simulink model "Feeder_1"  (Simulink 8.8)
settings: Solver=ode4  StartTime=0.0  StopTime=inf  FixedStep=Ts  RelTol=1e-3  EnableMultiTasking=on
PreLoadFcn:
  | Ts=125e-6;Core_Num = 0; np=1; nq=1; Vmin=.9;
PostLoadFcn:
  | Ts=125e-6;Core_Num = 0; np=1; nq=1; Vmin=.9;
InitFcn:
  | Ts=125e-6;Core_Num = 0; np=1; nq=1; Vmin=.9;
undefined symbols (not defined in the file or in its folder): another_event_name, DiscIntNeverNeededParam, I, j, Left, my_event_name, Right, type, V, X
libraries: powerlib x316, powerlib_meascontrol x227, simulink_extras x78, simulink x25, rtio_generic_c37_118 x22, ssn_lib x9, rtlab x6, powerlib_extras x3, artemis x1, rtio_opalrt_ml605ex1 x1, rtio_spectracom x1, rtio_generic_ethernet x1
(part 6 of 14)

== system Feeder_1/SM_NG/Single-Phase Dynamic Load43/model ==
  v : Inport
  PQ : Inport  Port=2
  -Q : Gain  SaturateOnIntegerOverflow=on  OutDataTypeStr=Inherit: Same as input  ParamDataTypeStr=Inherit: Same as input
  Break  Alg. Loop1 : Subsystem
  Complex to Magnitude-Angle : ComplexToMagnitudeAngle
  Complex to Real-Imag1 : ComplexToRealImag
  Constant : Constant
  Demux : Demux  Outputs=2
  Divide : Product  Inputs=**
  Gain : Gain  Gain=1.0114
  IC1 : InitialCondition
  IC2 : InitialCondition
  Magnitude-Angle to Complex : MagnitudeAngleToComplex
  PLL : Subsystem  mask{freq=fnom}
      mask prompts: freq "Initial frequency (Hz)"
  Positive Sequence  current : Subsystem
  RMS1 : powerlib_meascontrol/Measurements/RMS  TrueRMS=on  Freq=fnom  RMSInit=1  Ts=0
  Real-Imag to Complex : RealImagToComplex
  Real-Imag to Complex1 : RealImagToComplex
  Sum : Sum
  Transfer Fcn1 : TransferFcn  Numerator=[1 290.1]  Denominator=[1 298.8]
  Trigonometric Function1 : Trigonometry
  V> pu : Gain  Gain=1/Vbase/sqrt(3)  SaturateOnIntegerOverflow=on  OutDataTypeStr=Inherit: Same as input  ParamDataTypeStr=Inherit: Same as input
  V> pu1 : Gain  Gain=sqrt(2)  SaturateOnIntegerOverflow=on  OutDataTypeStr=Inherit: Same as input  ParamDataTypeStr=Inherit: Same as input
  i : Outport
  wires:
  V> pu/1 -> PLL/1(v (pu)), V> pu1/1
  Real-Imag to Complex/1 -> Positive Sequence  current/1(V1(pu))
  PQ/1 -> Demux/1
  Demux/1 -> Real-Imag to Complex1/1
  Demux/2 -> -Q/1
  Real-Imag to Complex1/1 -> Positive Sequence  current/2(S_ext)
  Complex to Real-Imag1/1 -> Real-Imag to Complex/1
  Complex to Real-Imag1/2 -> Real-Imag to Complex/2
  Magnitude-Angle to Complex/1 -> Complex to Real-Imag1/1
  Constant/1 -> PLL/2(freq (pu))
  PLL/1(alpha (rad)) -> Magnitude-Angle to Complex/2
  Complex to Magnitude-Angle/2 -> Sum/2
  PLL/2(wt) -> Sum/1
  Sum/1 -> Trigonometric Function1/1
  Trigonometric Function1/1 -> Divide/2
  Complex to Magnitude-Angle/1 -> Divide/1
  RMS1/1 -> IC1/1
  V> pu1/1 -> RMS1/1
  v/1 -> IC2/1
  Positive Sequence  current/1(I1(A)) -> Break  Alg. Loop1/1(In)
  Break  Alg. Loop1/1(Out) -> Complex to Magnitude-Angle/1
  IC1/1 -> Magnitude-Angle to Complex/1
  IC2/1 -> V> pu/1
  Transfer Fcn1/1 -> Gain/1
  Gain/1 -> i/1
  Divide/1 -> Transfer Fcn1/1
  -Q/1 -> Real-Imag to Complex1/2

== system Feeder_1/SM_NG/Single-Phase Dynamic Load44/model ==
  v : Inport
  PQ : Inport  Port=2
  -Q : Gain  SaturateOnIntegerOverflow=on  OutDataTypeStr=Inherit: Same as input  ParamDataTypeStr=Inherit: Same as input
  Break  Alg. Loop1 : Subsystem
  Complex to Magnitude-Angle : ComplexToMagnitudeAngle
  Complex to Real-Imag1 : ComplexToRealImag
  Constant : Constant
  Demux : Demux  Outputs=2
  Divide : Product  Inputs=**
  Gain : Gain  Gain=1.0114
  IC1 : InitialCondition
  IC2 : InitialCondition
  Magnitude-Angle to Complex : MagnitudeAngleToComplex
  PLL : Subsystem  mask{freq=fnom}
      mask prompts: freq "Initial frequency (Hz)"
  Positive Sequence  current : Subsystem
  RMS1 : powerlib_meascontrol/Measurements/RMS  TrueRMS=on  Freq=fnom  RMSInit=1  Ts=0
  Real-Imag to Complex : RealImagToComplex
  Real-Imag to Complex1 : RealImagToComplex
  Sum : Sum
  Transfer Fcn1 : TransferFcn  Numerator=[1 290.1]  Denominator=[1 298.8]
  Trigonometric Function1 : Trigonometry
  V> pu : Gain  Gain=1/Vbase/sqrt(3)  SaturateOnIntegerOverflow=on  OutDataTypeStr=Inherit: Same as input  ParamDataTypeStr=Inherit: Same as input
  V> pu1 : Gain  Gain=sqrt(2)  SaturateOnIntegerOverflow=on  OutDataTypeStr=Inherit: Same as input  ParamDataTypeStr=Inherit: Same as input
  i : Outport
  wires:
  V> pu/1 -> PLL/1(v (pu)), V> pu1/1
  Real-Imag to Complex/1 -> Positive Sequence  current/1(V1(pu))
  PQ/1 -> Demux/1
  Demux/1 -> Real-Imag to Complex1/1
  Demux/2 -> -Q/1
  Real-Imag to Complex1/1 -> Positive Sequence  current/2(S_ext)
  Complex to Real-Imag1/1 -> Real-Imag to Complex/1
  Complex to Real-Imag1/2 -> Real-Imag to Complex/2
  Magnitude-Angle to Complex/1 -> Complex to Real-Imag1/1
  Constant/1 -> PLL/2(freq (pu))
  PLL/1(alpha (rad)) -> Magnitude-Angle to Complex/2
  Complex to Magnitude-Angle/2 -> Sum/2
  PLL/2(wt) -> Sum/1
  Sum/1 -> Trigonometric Function1/1
  Trigonometric Function1/1 -> Divide/2
  Complex to Magnitude-Angle/1 -> Divide/1
  RMS1/1 -> IC1/1
  V> pu1/1 -> RMS1/1
  v/1 -> IC2/1
  Positive Sequence  current/1(I1(A)) -> Break  Alg. Loop1/1(In)
  Break  Alg. Loop1/1(Out) -> Complex to Magnitude-Angle/1
  IC1/1 -> Magnitude-Angle to Complex/1
  IC2/1 -> V> pu/1
  Transfer Fcn1/1 -> Gain/1
  Gain/1 -> i/1
  Divide/1 -> Transfer Fcn1/1
  -Q/1 -> Real-Imag to Complex1/2

== system Feeder_1/SM_NG/Single-Phase Dynamic Load45/model ==
  v : Inport
  PQ : Inport  Port=2
  -Q : Gain  SaturateOnIntegerOverflow=on  OutDataTypeStr=Inherit: Same as input  ParamDataTypeStr=Inherit: Same as input
  Break  Alg. Loop1 : Subsystem
  Complex to Magnitude-Angle : ComplexToMagnitudeAngle
  Complex to Real-Imag1 : ComplexToRealImag
  Constant : Constant
  Demux : Demux  Outputs=2
  Divide : Product  Inputs=**
  Gain : Gain  Gain=1.0114
  IC1 : InitialCondition
  IC2 : InitialCondition
  Magnitude-Angle to Complex : MagnitudeAngleToComplex
  PLL : Subsystem  mask{freq=fnom}
      mask prompts: freq "Initial frequency (Hz)"
  Positive Sequence  current : Subsystem
  RMS1 : powerlib_meascontrol/Measurements/RMS  TrueRMS=on  Freq=fnom  RMSInit=1  Ts=0
  Real-Imag to Complex : RealImagToComplex
  Real-Imag to Complex1 : RealImagToComplex
  Sum : Sum
  Transfer Fcn1 : TransferFcn  Numerator=[1 290.1]  Denominator=[1 298.8]
  Trigonometric Function1 : Trigonometry
  V> pu : Gain  Gain=1/Vbase/sqrt(3)  SaturateOnIntegerOverflow=on  OutDataTypeStr=Inherit: Same as input  ParamDataTypeStr=Inherit: Same as input
  V> pu1 : Gain  Gain=sqrt(2)  SaturateOnIntegerOverflow=on  OutDataTypeStr=Inherit: Same as input  ParamDataTypeStr=Inherit: Same as input
  i : Outport
  wires:
  V> pu/1 -> PLL/1(v (pu)), V> pu1/1
  Real-Imag to Complex/1 -> Positive Sequence  current/1(V1(pu))
  PQ/1 -> Demux/1
  Demux/1 -> Real-Imag to Complex1/1
  Demux/2 -> -Q/1
  Real-Imag to Complex1/1 -> Positive Sequence  current/2(S_ext)
  Complex to Real-Imag1/1 -> Real-Imag to Complex/1
  Complex to Real-Imag1/2 -> Real-Imag to Complex/2
  Magnitude-Angle to Complex/1 -> Complex to Real-Imag1/1
  Constant/1 -> PLL/2(freq (pu))
  PLL/1(alpha (rad)) -> Magnitude-Angle to Complex/2
  Complex to Magnitude-Angle/2 -> Sum/2
  PLL/2(wt) -> Sum/1
  Sum/1 -> Trigonometric Function1/1
  Trigonometric Function1/1 -> Divide/2
  Complex to Magnitude-Angle/1 -> Divide/1
  RMS1/1 -> IC1/1
  V> pu1/1 -> RMS1/1
  v/1 -> IC2/1
  Positive Sequence  current/1(I1(A)) -> Break  Alg. Loop1/1(In)
  Break  Alg. Loop1/1(Out) -> Complex to Magnitude-Angle/1
  IC1/1 -> Magnitude-Angle to Complex/1
  IC2/1 -> V> pu/1
  Transfer Fcn1/1 -> Gain/1
  Gain/1 -> i/1
  Divide/1 -> Transfer Fcn1/1
  -Q/1 -> Real-Imag to Complex1/2

== system Feeder_1/SM_NG/Single-Phase Dynamic Load46/model ==
  v : Inport
  PQ : Inport  Port=2
  -Q : Gain  SaturateOnIntegerOverflow=on  OutDataTypeStr=Inherit: Same as input  ParamDataTypeStr=Inherit: Same as input
  Break  Alg. Loop1 : Subsystem
  Complex to Magnitude-Angle : ComplexToMagnitudeAngle
  Complex to Real-Imag1 : ComplexToRealImag
  Constant : Constant
  Demux : Demux  Outputs=2
  Divide : Product  Inputs=**
  Gain : Gain  Gain=1.0114
  IC1 : InitialCondition
  IC2 : InitialCondition
  Magnitude-Angle to Complex : MagnitudeAngleToComplex
  PLL : Subsystem  mask{freq=fnom}
      mask prompts: freq "Initial frequency (Hz)"
  Positive Sequence  current : Subsystem
  RMS1 : powerlib_meascontrol/Measurements/RMS  TrueRMS=on  Freq=fnom  RMSInit=1  Ts=0
  Real-Imag to Complex : RealImagToComplex
  Real-Imag to Complex1 : RealImagToComplex
  Sum : Sum
  Transfer Fcn1 : TransferFcn  Numerator=[1 290.1]  Denominator=[1 298.8]
  Trigonometric Function1 : Trigonometry
  V> pu : Gain  Gain=1/Vbase/sqrt(3)  SaturateOnIntegerOverflow=on  OutDataTypeStr=Inherit: Same as input  ParamDataTypeStr=Inherit: Same as input
  V> pu1 : Gain  Gain=sqrt(2)  SaturateOnIntegerOverflow=on  OutDataTypeStr=Inherit: Same as input  ParamDataTypeStr=Inherit: Same as input
  i : Outport
  wires:
  V> pu/1 -> PLL/1(v (pu)), V> pu1/1
  Real-Imag to Complex/1 -> Positive Sequence  current/1(V1(pu))
  PQ/1 -> Demux/1
  Demux/1 -> Real-Imag to Complex1/1
  Demux/2 -> -Q/1
  Real-Imag to Complex1/1 -> Positive Sequence  current/2(S_ext)
  Complex to Real-Imag1/1 -> Real-Imag to Complex/1
  Complex to Real-Imag1/2 -> Real-Imag to Complex/2
  Magnitude-Angle to Complex/1 -> Complex to Real-Imag1/1
  Constant/1 -> PLL/2(freq (pu))
  PLL/1(alpha (rad)) -> Magnitude-Angle to Complex/2
  Complex to Magnitude-Angle/2 -> Sum/2
  PLL/2(wt) -> Sum/1
  Sum/1 -> Trigonometric Function1/1
  Trigonometric Function1/1 -> Divide/2
  Complex to Magnitude-Angle/1 -> Divide/1
  RMS1/1 -> IC1/1
  V> pu1/1 -> RMS1/1
  v/1 -> IC2/1
  Positive Sequence  current/1(I1(A)) -> Break  Alg. Loop1/1(In)
  Break  Alg. Loop1/1(Out) -> Complex to Magnitude-Angle/1
  IC1/1 -> Magnitude-Angle to Complex/1
  IC2/1 -> V> pu/1
  Transfer Fcn1/1 -> Gain/1
  Gain/1 -> i/1
  Divide/1 -> Transfer Fcn1/1
  -Q/1 -> Real-Imag to Complex1/2

== system Feeder_1/SM_NG/Single-Phase Dynamic Load47/model ==
  v : Inport
  PQ : Inport  Port=2
  -Q : Gain  SaturateOnIntegerOverflow=on  OutDataTypeStr=Inherit: Same as input  ParamDataTypeStr=Inherit: Same as input
  Break  Alg. Loop1 : Subsystem
  Complex to Magnitude-Angle : ComplexToMagnitudeAngle
  Complex to Real-Imag1 : ComplexToRealImag
  Constant : Constant
  Demux : Demux  Outputs=2
  Divide : Product  Inputs=**
  Gain : Gain  Gain=1.0114
  IC1 : InitialCondition
  IC2 : InitialCondition
  Magnitude-Angle to Complex : MagnitudeAngleToComplex
  PLL : Subsystem  mask{freq=fnom}
      mask prompts: freq "Initial frequency (Hz)"
  Positive Sequence  current : Subsystem
  RMS1 : powerlib_meascontrol/Measurements/RMS  TrueRMS=on  Freq=fnom  RMSInit=1  Ts=0
  Real-Imag to Complex : RealImagToComplex
  Real-Imag to Complex1 : RealImagToComplex
  Sum : Sum
  Transfer Fcn1 : TransferFcn  Numerator=[1 290.1]  Denominator=[1 298.8]
  Trigonometric Function1 : Trigonometry
  V> pu : Gain  Gain=1/Vbase/sqrt(3)  SaturateOnIntegerOverflow=on  OutDataTypeStr=Inherit: Same as input  ParamDataTypeStr=Inherit: Same as input
  V> pu1 : Gain  Gain=sqrt(2)  SaturateOnIntegerOverflow=on  OutDataTypeStr=Inherit: Same as input  ParamDataTypeStr=Inherit: Same as input
  i : Outport
  wires:
  V> pu/1 -> PLL/1(v (pu)), V> pu1/1
  Real-Imag to Complex/1 -> Positive Sequence  current/1(V1(pu))
  PQ/1 -> Demux/1
  Demux/1 -> Real-Imag to Complex1/1
  Demux/2 -> -Q/1
  Real-Imag to Complex1/1 -> Positive Sequence  current/2(S_ext)
  Complex to Real-Imag1/1 -> Real-Imag to Complex/1
  Complex to Real-Imag1/2 -> Real-Imag to Complex/2
  Magnitude-Angle to Complex/1 -> Complex to Real-Imag1/1
  Constant/1 -> PLL/2(freq (pu))
  PLL/1(alpha (rad)) -> Magnitude-Angle to Complex/2
  Complex to Magnitude-Angle/2 -> Sum/2
  PLL/2(wt) -> Sum/1
  Sum/1 -> Trigonometric Function1/1
  Trigonometric Function1/1 -> Divide/2
  Complex to Magnitude-Angle/1 -> Divide/1
  RMS1/1 -> IC1/1
  V> pu1/1 -> RMS1/1
  v/1 -> IC2/1
  Positive Sequence  current/1(I1(A)) -> Break  Alg. Loop1/1(In)
  Break  Alg. Loop1/1(Out) -> Complex to Magnitude-Angle/1
  IC1/1 -> Magnitude-Angle to Complex/1
  IC2/1 -> V> pu/1
  Transfer Fcn1/1 -> Gain/1
  Gain/1 -> i/1
  Divide/1 -> Transfer Fcn1/1
  -Q/1 -> Real-Imag to Complex1/2

== system Feeder_1/SM_NG/Single-Phase Dynamic Load48/model ==
  v : Inport
  PQ : Inport  Port=2
  -Q : Gain  SaturateOnIntegerOverflow=on  OutDataTypeStr=Inherit: Same as input  ParamDataTypeStr=Inherit: Same as input
  Break  Alg. Loop1 : Subsystem
  Complex to Magnitude-Angle : ComplexToMagnitudeAngle
  Complex to Real-Imag1 : ComplexToRealImag
  Constant : Constant
  Demux : Demux  Outputs=2
  Divide : Product  Inputs=**
  Gain : Gain  Gain=1.0114
  IC1 : InitialCondition
  IC2 : InitialCondition
  Magnitude-Angle to Complex : MagnitudeAngleToComplex
  PLL : Subsystem  mask{freq=fnom}
      mask prompts: freq "Initial frequency (Hz)"
  Positive Sequence  current : Subsystem
  RMS1 : powerlib_meascontrol/Measurements/RMS  TrueRMS=on  Freq=fnom  RMSInit=1  Ts=0
  Real-Imag to Complex : RealImagToComplex
  Real-Imag to Complex1 : RealImagToComplex
  Sum : Sum
  Transfer Fcn1 : TransferFcn  Numerator=[1 290.1]  Denominator=[1 298.8]
  Trigonometric Function1 : Trigonometry
  V> pu : Gain  Gain=1/Vbase/sqrt(3)  SaturateOnIntegerOverflow=on  OutDataTypeStr=Inherit: Same as input  ParamDataTypeStr=Inherit: Same as input
  V> pu1 : Gain  Gain=sqrt(2)  SaturateOnIntegerOverflow=on  OutDataTypeStr=Inherit: Same as input  ParamDataTypeStr=Inherit: Same as input
  i : Outport
  wires:
  V> pu/1 -> PLL/1(v (pu)), V> pu1/1
  Real-Imag to Complex/1 -> Positive Sequence  current/1(V1(pu))
  PQ/1 -> Demux/1
  Demux/1 -> Real-Imag to Complex1/1
  Demux/2 -> -Q/1
  Real-Imag to Complex1/1 -> Positive Sequence  current/2(S_ext)
  Complex to Real-Imag1/1 -> Real-Imag to Complex/1
  Complex to Real-Imag1/2 -> Real-Imag to Complex/2
  Magnitude-Angle to Complex/1 -> Complex to Real-Imag1/1
  Constant/1 -> PLL/2(freq (pu))
  PLL/1(alpha (rad)) -> Magnitude-Angle to Complex/2
  Complex to Magnitude-Angle/2 -> Sum/2
  PLL/2(wt) -> Sum/1
  Sum/1 -> Trigonometric Function1/1
  Trigonometric Function1/1 -> Divide/2
  Complex to Magnitude-Angle/1 -> Divide/1
  RMS1/1 -> IC1/1
  V> pu1/1 -> RMS1/1
  v/1 -> IC2/1
  Positive Sequence  current/1(I1(A)) -> Break  Alg. Loop1/1(In)
  Break  Alg. Loop1/1(Out) -> Complex to Magnitude-Angle/1
  IC1/1 -> Magnitude-Angle to Complex/1
  IC2/1 -> V> pu/1
  Transfer Fcn1/1 -> Gain/1
  Gain/1 -> i/1
  Divide/1 -> Transfer Fcn1/1
  -Q/1 -> Real-Imag to Complex1/2

== system Feeder_1/SM_NG/Single-Phase Dynamic Load49/model ==
  v : Inport
  PQ : Inport  Port=2
  -Q : Gain  SaturateOnIntegerOverflow=on  OutDataTypeStr=Inherit: Same as input  ParamDataTypeStr=Inherit: Same as input
  Break  Alg. Loop1 : Subsystem
  Complex to Magnitude-Angle : ComplexToMagnitudeAngle
  Complex to Real-Imag1 : ComplexToRealImag
  Constant : Constant
  Demux : Demux  Outputs=2
  Divide : Product  Inputs=**
  Gain : Gain  Gain=1.0114
  IC1 : InitialCondition
  IC2 : InitialCondition
  Magnitude-Angle to Complex : MagnitudeAngleToComplex
  PLL : Subsystem  mask{freq=fnom}
      mask prompts: freq "Initial frequency (Hz)"
  Positive Sequence  current : Subsystem
  RMS1 : powerlib_meascontrol/Measurements/RMS  TrueRMS=on  Freq=fnom  RMSInit=1  Ts=0
  Real-Imag to Complex : RealImagToComplex
  Real-Imag to Complex1 : RealImagToComplex
  Sum : Sum
  Transfer Fcn1 : TransferFcn  Numerator=[1 290.1]  Denominator=[1 298.8]
  Trigonometric Function1 : Trigonometry
  V> pu : Gain  Gain=1/Vbase/sqrt(3)  SaturateOnIntegerOverflow=on  OutDataTypeStr=Inherit: Same as input  ParamDataTypeStr=Inherit: Same as input
  V> pu1 : Gain  Gain=sqrt(2)  SaturateOnIntegerOverflow=on  OutDataTypeStr=Inherit: Same as input  ParamDataTypeStr=Inherit: Same as input
  i : Outport
  wires:
  V> pu/1 -> PLL/1(v (pu)), V> pu1/1
  Real-Imag to Complex/1 -> Positive Sequence  current/1(V1(pu))
  PQ/1 -> Demux/1
  Demux/1 -> Real-Imag to Complex1/1
  Demux/2 -> -Q/1
  Real-Imag to Complex1/1 -> Positive Sequence  current/2(S_ext)
  Complex to Real-Imag1/1 -> Real-Imag to Complex/1
  Complex to Real-Imag1/2 -> Real-Imag to Complex/2
  Magnitude-Angle to Complex/1 -> Complex to Real-Imag1/1
  Constant/1 -> PLL/2(freq (pu))
  PLL/1(alpha (rad)) -> Magnitude-Angle to Complex/2
  Complex to Magnitude-Angle/2 -> Sum/2
  PLL/2(wt) -> Sum/1
  Sum/1 -> Trigonometric Function1/1
  Trigonometric Function1/1 -> Divide/2
  Complex to Magnitude-Angle/1 -> Divide/1
  RMS1/1 -> IC1/1
  V> pu1/1 -> RMS1/1
  v/1 -> IC2/1
  Positive Sequence  current/1(I1(A)) -> Break  Alg. Loop1/1(In)
  Break  Alg. Loop1/1(Out) -> Complex to Magnitude-Angle/1
  IC1/1 -> Magnitude-Angle to Complex/1
  IC2/1 -> V> pu/1
  Transfer Fcn1/1 -> Gain/1
  Gain/1 -> i/1
  Divide/1 -> Transfer Fcn1/1
  -Q/1 -> Real-Imag to Complex1/2

== system Feeder_1/SM_NG/Single-Phase Dynamic Load50/model ==
  v : Inport
  PQ : Inport  Port=2
  -Q : Gain  SaturateOnIntegerOverflow=on  OutDataTypeStr=Inherit: Same as input  ParamDataTypeStr=Inherit: Same as input
  Break  Alg. Loop1 : Subsystem
  Complex to Magnitude-Angle : ComplexToMagnitudeAngle
  Complex to Real-Imag1 : ComplexToRealImag
  Constant : Constant
  Demux : Demux  Outputs=2
  Divide : Product  Inputs=**
  Gain : Gain  Gain=1.0114
  IC1 : InitialCondition
  IC2 : InitialCondition
  Magnitude-Angle to Complex : MagnitudeAngleToComplex
  PLL : Subsystem  mask{freq=fnom}
      mask prompts: freq "Initial frequency (Hz)"
  Positive Sequence  current : Subsystem
  RMS1 : powerlib_meascontrol/Measurements/RMS  TrueRMS=on  Freq=fnom  RMSInit=1  Ts=0
  Real-Imag to Complex : RealImagToComplex
  Real-Imag to Complex1 : RealImagToComplex
  Sum : Sum
  Transfer Fcn1 : TransferFcn  Numerator=[1 290.1]  Denominator=[1 298.8]
  Trigonometric Function1 : Trigonometry
  V> pu : Gain  Gain=1/Vbase/sqrt(3)  SaturateOnIntegerOverflow=on  OutDataTypeStr=Inherit: Same as input  ParamDataTypeStr=Inherit: Same as input
  V> pu1 : Gain  Gain=sqrt(2)  SaturateOnIntegerOverflow=on  OutDataTypeStr=Inherit: Same as input  ParamDataTypeStr=Inherit: Same as input
  i : Outport
  wires:
  V> pu/1 -> PLL/1(v (pu)), V> pu1/1
  Real-Imag to Complex/1 -> Positive Sequence  current/1(V1(pu))
  PQ/1 -> Demux/1
  Demux/1 -> Real-Imag to Complex1/1
  Demux/2 -> -Q/1
  Real-Imag to Complex1/1 -> Positive Sequence  current/2(S_ext)
  Complex to Real-Imag1/1 -> Real-Imag to Complex/1
  Complex to Real-Imag1/2 -> Real-Imag to Complex/2
  Magnitude-Angle to Complex/1 -> Complex to Real-Imag1/1
  Constant/1 -> PLL/2(freq (pu))
  PLL/1(alpha (rad)) -> Magnitude-Angle to Complex/2
  Complex to Magnitude-Angle/2 -> Sum/2
  PLL/2(wt) -> Sum/1
  Sum/1 -> Trigonometric Function1/1
  Trigonometric Function1/1 -> Divide/2
  Complex to Magnitude-Angle/1 -> Divide/1
  RMS1/1 -> IC1/1
  V> pu1/1 -> RMS1/1
  v/1 -> IC2/1
  Positive Sequence  current/1(I1(A)) -> Break  Alg. Loop1/1(In)
  Break  Alg. Loop1/1(Out) -> Complex to Magnitude-Angle/1
  IC1/1 -> Magnitude-Angle to Complex/1
  IC2/1 -> V> pu/1
  Transfer Fcn1/1 -> Gain/1
  Gain/1 -> i/1
  Divide/1 -> Transfer Fcn1/1
  -Q/1 -> Real-Imag to Complex1/2

== system Feeder_1/SM_NG/Single-Phase Dynamic Load51/model ==
  v : Inport
  PQ : Inport  Port=2
  -Q : Gain  SaturateOnIntegerOverflow=on  OutDataTypeStr=Inherit: Same as input  ParamDataTypeStr=Inherit: Same as input
  Break  Alg. Loop1 : Subsystem
  Complex to Magnitude-Angle : ComplexToMagnitudeAngle
  Complex to Real-Imag1 : ComplexToRealImag
  Constant : Constant
  Demux : Demux  Outputs=2
  Divide : Product  Inputs=**
  Gain : Gain  Gain=1.0114
  IC1 : InitialCondition
  IC2 : InitialCondition
  Magnitude-Angle to Complex : MagnitudeAngleToComplex
  PLL : Subsystem  mask{freq=fnom}
      mask prompts: freq "Initial frequency (Hz)"
  Positive Sequence  current : Subsystem
  RMS1 : powerlib_meascontrol/Measurements/RMS  TrueRMS=on  Freq=fnom  RMSInit=1  Ts=0
  Real-Imag to Complex : RealImagToComplex
  Real-Imag to Complex1 : RealImagToComplex
  Sum : Sum
  Transfer Fcn1 : TransferFcn  Numerator=[1 290.1]  Denominator=[1 298.8]
  Trigonometric Function1 : Trigonometry
  V> pu : Gain  Gain=1/Vbase/sqrt(3)  SaturateOnIntegerOverflow=on  OutDataTypeStr=Inherit: Same as input  ParamDataTypeStr=Inherit: Same as input
  V> pu1 : Gain  Gain=sqrt(2)  SaturateOnIntegerOverflow=on  OutDataTypeStr=Inherit: Same as input  ParamDataTypeStr=Inherit: Same as input
  i : Outport
  wires:
  V> pu/1 -> PLL/1(v (pu)), V> pu1/1
  Real-Imag to Complex/1 -> Positive Sequence  current/1(V1(pu))
  PQ/1 -> Demux/1
  Demux/1 -> Real-Imag to Complex1/1
  Demux/2 -> -Q/1
  Real-Imag to Complex1/1 -> Positive Sequence  current/2(S_ext)
  Complex to Real-Imag1/1 -> Real-Imag to Complex/1
  Complex to Real-Imag1/2 -> Real-Imag to Complex/2
  Magnitude-Angle to Complex/1 -> Complex to Real-Imag1/1
  Constant/1 -> PLL/2(freq (pu))
  PLL/1(alpha (rad)) -> Magnitude-Angle to Complex/2
  Complex to Magnitude-Angle/2 -> Sum/2
  PLL/2(wt) -> Sum/1
  Sum/1 -> Trigonometric Function1/1
  Trigonometric Function1/1 -> Divide/2
  Complex to Magnitude-Angle/1 -> Divide/1
  RMS1/1 -> IC1/1
  V> pu1/1 -> RMS1/1
  v/1 -> IC2/1
  Positive Sequence  current/1(I1(A)) -> Break  Alg. Loop1/1(In)
  Break  Alg. Loop1/1(Out) -> Complex to Magnitude-Angle/1
  IC1/1 -> Magnitude-Angle to Complex/1
  IC2/1 -> V> pu/1
  Transfer Fcn1/1 -> Gain/1
  Gain/1 -> i/1
  Divide/1 -> Transfer Fcn1/1
  -Q/1 -> Real-Imag to Complex1/2

== system Feeder_1/SM_NG/Single-Phase Dynamic Load52/model ==
  v : Inport
  PQ : Inport  Port=2
  -Q : Gain  SaturateOnIntegerOverflow=on  OutDataTypeStr=Inherit: Same as input  ParamDataTypeStr=Inherit: Same as input
  Break  Alg. Loop1 : Subsystem
  Complex to Magnitude-Angle : ComplexToMagnitudeAngle
  Complex to Real-Imag1 : ComplexToRealImag
  Constant : Constant
  Demux : Demux  Outputs=2
  Divide : Product  Inputs=**
  Gain : Gain  Gain=1.0114
  IC1 : InitialCondition
  IC2 : InitialCondition
  Magnitude-Angle to Complex : MagnitudeAngleToComplex
  PLL : Subsystem  mask{freq=fnom}
      mask prompts: freq "Initial frequency (Hz)"
  Positive Sequence  current : Subsystem
  RMS1 : powerlib_meascontrol/Measurements/RMS  TrueRMS=on  Freq=fnom  RMSInit=1  Ts=0
  Real-Imag to Complex : RealImagToComplex
  Real-Imag to Complex1 : RealImagToComplex
  Sum : Sum
  Transfer Fcn1 : TransferFcn  Numerator=[1 290.1]  Denominator=[1 298.8]
  Trigonometric Function1 : Trigonometry
  V> pu : Gain  Gain=1/Vbase/sqrt(3)  SaturateOnIntegerOverflow=on  OutDataTypeStr=Inherit: Same as input  ParamDataTypeStr=Inherit: Same as input
  V> pu1 : Gain  Gain=sqrt(2)  SaturateOnIntegerOverflow=on  OutDataTypeStr=Inherit: Same as input  ParamDataTypeStr=Inherit: Same as input
  i : Outport
  wires:
  V> pu/1 -> PLL/1(v (pu)), V> pu1/1
  Real-Imag to Complex/1 -> Positive Sequence  current/1(V1(pu))
  PQ/1 -> Demux/1
  Demux/1 -> Real-Imag to Complex1/1
  Demux/2 -> -Q/1
  Real-Imag to Complex1/1 -> Positive Sequence  current/2(S_ext)
  Complex to Real-Imag1/1 -> Real-Imag to Complex/1
  Complex to Real-Imag1/2 -> Real-Imag to Complex/2
  Magnitude-Angle to Complex/1 -> Complex to Real-Imag1/1
  Constant/1 -> PLL/2(freq (pu))
  PLL/1(alpha (rad)) -> Magnitude-Angle to Complex/2
  Complex to Magnitude-Angle/2 -> Sum/2
  PLL/2(wt) -> Sum/1
  Sum/1 -> Trigonometric Function1/1
  Trigonometric Function1/1 -> Divide/2
  Complex to Magnitude-Angle/1 -> Divide/1
  RMS1/1 -> IC1/1
  V> pu1/1 -> RMS1/1
  v/1 -> IC2/1
  Positive Sequence  current/1(I1(A)) -> Break  Alg. Loop1/1(In)
  Break  Alg. Loop1/1(Out) -> Complex to Magnitude-Angle/1
  IC1/1 -> Magnitude-Angle to Complex/1
  IC2/1 -> V> pu/1
  Transfer Fcn1/1 -> Gain/1
  Gain/1 -> i/1
  Divide/1 -> Transfer Fcn1/1
  -Q/1 -> Real-Imag to Complex1/2

== system Feeder_1/SM_NG/Single-Phase Dynamic Load53/model ==
  v : Inport
  PQ : Inport  Port=2
  -Q : Gain  SaturateOnIntegerOverflow=on  OutDataTypeStr=Inherit: Same as input  ParamDataTypeStr=Inherit: Same as input
  Break  Alg. Loop1 : Subsystem
  Complex to Magnitude-Angle : ComplexToMagnitudeAngle
  Complex to Real-Imag1 : ComplexToRealImag
  Constant : Constant
  Demux : Demux  Outputs=2
  Divide : Product  Inputs=**
  Gain : Gain  Gain=1.0114
  IC1 : InitialCondition
  IC2 : InitialCondition
  Magnitude-Angle to Complex : MagnitudeAngleToComplex
  PLL : Subsystem  mask{freq=fnom}
      mask prompts: freq "Initial frequency (Hz)"
  Positive Sequence  current : Subsystem
  RMS1 : powerlib_meascontrol/Measurements/RMS  TrueRMS=on  Freq=fnom  RMSInit=1  Ts=0
  Real-Imag to Complex : RealImagToComplex
  Real-Imag to Complex1 : RealImagToComplex
  Sum : Sum
  Transfer Fcn1 : TransferFcn  Numerator=[1 290.1]  Denominator=[1 298.8]
  Trigonometric Function1 : Trigonometry
  V> pu : Gain  Gain=1/Vbase/sqrt(3)  SaturateOnIntegerOverflow=on  OutDataTypeStr=Inherit: Same as input  ParamDataTypeStr=Inherit: Same as input
  V> pu1 : Gain  Gain=sqrt(2)  SaturateOnIntegerOverflow=on  OutDataTypeStr=Inherit: Same as input  ParamDataTypeStr=Inherit: Same as input
  i : Outport
  wires:
  V> pu/1 -> PLL/1(v (pu)), V> pu1/1
  Real-Imag to Complex/1 -> Positive Sequence  current/1(V1(pu))
  PQ/1 -> Demux/1
  Demux/1 -> Real-Imag to Complex1/1
  Demux/2 -> -Q/1
  Real-Imag to Complex1/1 -> Positive Sequence  current/2(S_ext)
  Complex to Real-Imag1/1 -> Real-Imag to Complex/1
  Complex to Real-Imag1/2 -> Real-Imag to Complex/2
  Magnitude-Angle to Complex/1 -> Complex to Real-Imag1/1
  Constant/1 -> PLL/2(freq (pu))
  PLL/1(alpha (rad)) -> Magnitude-Angle to Complex/2
  Complex to Magnitude-Angle/2 -> Sum/2
  PLL/2(wt) -> Sum/1
  Sum/1 -> Trigonometric Function1/1
  Trigonometric Function1/1 -> Divide/2
  Complex to Magnitude-Angle/1 -> Divide/1
  RMS1/1 -> IC1/1
  V> pu1/1 -> RMS1/1
  v/1 -> IC2/1
  Positive Sequence  current/1(I1(A)) -> Break  Alg. Loop1/1(In)
  Break  Alg. Loop1/1(Out) -> Complex to Magnitude-Angle/1
  IC1/1 -> Magnitude-Angle to Complex/1
  IC2/1 -> V> pu/1
  Transfer Fcn1/1 -> Gain/1
  Gain/1 -> i/1
  Divide/1 -> Transfer Fcn1/1
  -Q/1 -> Real-Imag to Complex1/2

== system Feeder_1/SM_NG/Single-Phase Dynamic Load54/model ==
  v : Inport
  PQ : Inport  Port=2
  -Q : Gain  SaturateOnIntegerOverflow=on  OutDataTypeStr=Inherit: Same as input  ParamDataTypeStr=Inherit: Same as input
  Break  Alg. Loop1 : Subsystem
  Complex to Magnitude-Angle : ComplexToMagnitudeAngle
  Complex to Real-Imag1 : ComplexToRealImag
  Constant : Constant
  Demux : Demux  Outputs=2
  Divide : Product  Inputs=**
  Gain : Gain  Gain=1.0114
  IC1 : InitialCondition
  IC2 : InitialCondition
  Magnitude-Angle to Complex : MagnitudeAngleToComplex
  PLL : Subsystem  mask{freq=fnom}
      mask prompts: freq "Initial frequency (Hz)"
  Positive Sequence  current : Subsystem
  RMS1 : powerlib_meascontrol/Measurements/RMS  TrueRMS=on  Freq=fnom  RMSInit=1  Ts=0
  Real-Imag to Complex : RealImagToComplex
  Real-Imag to Complex1 : RealImagToComplex
  Sum : Sum
  Transfer Fcn1 : TransferFcn  Numerator=[1 290.1]  Denominator=[1 298.8]
  Trigonometric Function1 : Trigonometry
  V> pu : Gain  Gain=1/Vbase/sqrt(3)  SaturateOnIntegerOverflow=on  OutDataTypeStr=Inherit: Same as input  ParamDataTypeStr=Inherit: Same as input
  V> pu1 : Gain  Gain=sqrt(2)  SaturateOnIntegerOverflow=on  OutDataTypeStr=Inherit: Same as input  ParamDataTypeStr=Inherit: Same as input
  i : Outport
  wires:
  V> pu/1 -> PLL/1(v (pu)), V> pu1/1
  Real-Imag to Complex/1 -> Positive Sequence  current/1(V1(pu))
  PQ/1 -> Demux/1
  Demux/1 -> Real-Imag to Complex1/1
  Demux/2 -> -Q/1
  Real-Imag to Complex1/1 -> Positive Sequence  current/2(S_ext)
  Complex to Real-Imag1/1 -> Real-Imag to Complex/1
  Complex to Real-Imag1/2 -> Real-Imag to Complex/2
  Magnitude-Angle to Complex/1 -> Complex to Real-Imag1/1
  Constant/1 -> PLL/2(freq (pu))
  PLL/1(alpha (rad)) -> Magnitude-Angle to Complex/2
  Complex to Magnitude-Angle/2 -> Sum/2
  PLL/2(wt) -> Sum/1
  Sum/1 -> Trigonometric Function1/1
  Trigonometric Function1/1 -> Divide/2
  Complex to Magnitude-Angle/1 -> Divide/1
  RMS1/1 -> IC1/1
  V> pu1/1 -> RMS1/1
  v/1 -> IC2/1
  Positive Sequence  current/1(I1(A)) -> Break  Alg. Loop1/1(In)
  Break  Alg. Loop1/1(Out) -> Complex to Magnitude-Angle/1
  IC1/1 -> Magnitude-Angle to Complex/1
  IC2/1 -> V> pu/1
  Transfer Fcn1/1 -> Gain/1
  Gain/1 -> i/1
  Divide/1 -> Transfer Fcn1/1
  -Q/1 -> Real-Imag to Complex1/2

== system Feeder_1/SM_NG/Single-Phase Dynamic Load55/model ==
  v : Inport
  PQ : Inport  Port=2
  -Q : Gain  SaturateOnIntegerOverflow=on  OutDataTypeStr=Inherit: Same as input  ParamDataTypeStr=Inherit: Same as input
  Break  Alg. Loop1 : Subsystem
  Complex to Magnitude-Angle : ComplexToMagnitudeAngle
  Complex to Real-Imag1 : ComplexToRealImag
  Constant : Constant
  Demux : Demux  Outputs=2
  Divide : Product  Inputs=**
  Gain : Gain  Gain=1.0114
  IC1 : InitialCondition
  IC2 : InitialCondition
  Magnitude-Angle to Complex : MagnitudeAngleToComplex
  PLL : Subsystem  mask{freq=fnom}
      mask prompts: freq "Initial frequency (Hz)"
  Positive Sequence  current : Subsystem
  RMS1 : powerlib_meascontrol/Measurements/RMS  TrueRMS=on  Freq=fnom  RMSInit=1  Ts=0
  Real-Imag to Complex : RealImagToComplex
  Real-Imag to Complex1 : RealImagToComplex
  Sum : Sum
  Transfer Fcn1 : TransferFcn  Numerator=[1 290.1]  Denominator=[1 298.8]
  Trigonometric Function1 : Trigonometry
  V> pu : Gain  Gain=1/Vbase/sqrt(3)  SaturateOnIntegerOverflow=on  OutDataTypeStr=Inherit: Same as input  ParamDataTypeStr=Inherit: Same as input
  V> pu1 : Gain  Gain=sqrt(2)  SaturateOnIntegerOverflow=on  OutDataTypeStr=Inherit: Same as input  ParamDataTypeStr=Inherit: Same as input
  i : Outport
  wires:
  V> pu/1 -> PLL/1(v (pu)), V> pu1/1
  Real-Imag to Complex/1 -> Positive Sequence  current/1(V1(pu))
  PQ/1 -> Demux/1
  Demux/1 -> Real-Imag to Complex1/1
  Demux/2 -> -Q/1
  Real-Imag to Complex1/1 -> Positive Sequence  current/2(S_ext)
  Complex to Real-Imag1/1 -> Real-Imag to Complex/1
  Complex to Real-Imag1/2 -> Real-Imag to Complex/2
  Magnitude-Angle to Complex/1 -> Complex to Real-Imag1/1
  Constant/1 -> PLL/2(freq (pu))
  PLL/1(alpha (rad)) -> Magnitude-Angle to Complex/2
  Complex to Magnitude-Angle/2 -> Sum/2
  PLL/2(wt) -> Sum/1
  Sum/1 -> Trigonometric Function1/1
  Trigonometric Function1/1 -> Divide/2
  Complex to Magnitude-Angle/1 -> Divide/1
  RMS1/1 -> IC1/1
  V> pu1/1 -> RMS1/1
  v/1 -> IC2/1
  Positive Sequence  current/1(I1(A)) -> Break  Alg. Loop1/1(In)
  Break  Alg. Loop1/1(Out) -> Complex to Magnitude-Angle/1
  IC1/1 -> Magnitude-Angle to Complex/1
  IC2/1 -> V> pu/1
  Transfer Fcn1/1 -> Gain/1
  Gain/1 -> i/1
  Divide/1 -> Transfer Fcn1/1
  -Q/1 -> Real-Imag to Complex1/2

== system Feeder_1/SM_NG/Single-Phase Dynamic Load56/model ==
  v : Inport
  PQ : Inport  Port=2
  -Q : Gain  SaturateOnIntegerOverflow=on  OutDataTypeStr=Inherit: Same as input  ParamDataTypeStr=Inherit: Same as input
  Break  Alg. Loop1 : Subsystem
  Complex to Magnitude-Angle : ComplexToMagnitudeAngle
  Complex to Real-Imag1 : ComplexToRealImag
  Constant : Constant
  Demux : Demux  Outputs=2
  Divide : Product  Inputs=**
  Gain : Gain  Gain=1.0114
  IC1 : InitialCondition
  IC2 : InitialCondition
  Magnitude-Angle to Complex : MagnitudeAngleToComplex
  PLL : Subsystem  mask{freq=fnom}
      mask prompts: freq "Initial frequency (Hz)"
  Positive Sequence  current : Subsystem
  RMS1 : powerlib_meascontrol/Measurements/RMS  TrueRMS=on  Freq=fnom  RMSInit=1  Ts=0
  Real-Imag to Complex : RealImagToComplex
  Real-Imag to Complex1 : RealImagToComplex
  Sum : Sum
  Transfer Fcn1 : TransferFcn  Numerator=[1 290.1]  Denominator=[1 298.8]
  Trigonometric Function1 : Trigonometry
  V> pu : Gain  Gain=1/Vbase/sqrt(3)  SaturateOnIntegerOverflow=on  OutDataTypeStr=Inherit: Same as input  ParamDataTypeStr=Inherit: Same as input
  V> pu1 : Gain  Gain=sqrt(2)  SaturateOnIntegerOverflow=on  OutDataTypeStr=Inherit: Same as input  ParamDataTypeStr=Inherit: Same as input
  i : Outport
  wires:
  V> pu/1 -> PLL/1(v (pu)), V> pu1/1
  Real-Imag to Complex/1 -> Positive Sequence  current/1(V1(pu))
  PQ/1 -> Demux/1
  Demux/1 -> Real-Imag to Complex1/1
  Demux/2 -> -Q/1
  Real-Imag to Complex1/1 -> Positive Sequence  current/2(S_ext)
  Complex to Real-Imag1/1 -> Real-Imag to Complex/1
  Complex to Real-Imag1/2 -> Real-Imag to Complex/2
  Magnitude-Angle to Complex/1 -> Complex to Real-Imag1/1
  Constant/1 -> PLL/2(freq (pu))
  PLL/1(alpha (rad)) -> Magnitude-Angle to Complex/2
  Complex to Magnitude-Angle/2 -> Sum/2
  PLL/2(wt) -> Sum/1
  Sum/1 -> Trigonometric Function1/1
  Trigonometric Function1/1 -> Divide/2
  Complex to Magnitude-Angle/1 -> Divide/1
  RMS1/1 -> IC1/1
  V> pu1/1 -> RMS1/1
  v/1 -> IC2/1
  Positive Sequence  current/1(I1(A)) -> Break  Alg. Loop1/1(In)
  Break  Alg. Loop1/1(Out) -> Complex to Magnitude-Angle/1
  IC1/1 -> Magnitude-Angle to Complex/1
  IC2/1 -> V> pu/1
  Transfer Fcn1/1 -> Gain/1
  Gain/1 -> i/1
  Divide/1 -> Transfer Fcn1/1
  -Q/1 -> Real-Imag to Complex1/2

== system Feeder_1/SM_NG/Single-Phase Dynamic Load57/model ==
  v : Inport
  PQ : Inport  Port=2
  -Q : Gain  SaturateOnIntegerOverflow=on  OutDataTypeStr=Inherit: Same as input  ParamDataTypeStr=Inherit: Same as input
  Break  Alg. Loop1 : Subsystem
  Complex to Magnitude-Angle : ComplexToMagnitudeAngle
  Complex to Real-Imag1 : ComplexToRealImag
  Constant : Constant
  Demux : Demux  Outputs=2
  Divide : Product  Inputs=**
  Gain : Gain  Gain=1.0114
  IC1 : InitialCondition
  IC2 : InitialCondition
  Magnitude-Angle to Complex : MagnitudeAngleToComplex
  PLL : Subsystem  mask{freq=fnom}
      mask prompts: freq "Initial frequency (Hz)"
  Positive Sequence  current : Subsystem
  RMS1 : powerlib_meascontrol/Measurements/RMS  TrueRMS=on  Freq=fnom  RMSInit=1  Ts=0
  Real-Imag to Complex : RealImagToComplex
  Real-Imag to Complex1 : RealImagToComplex
  Sum : Sum
  Transfer Fcn1 : TransferFcn  Numerator=[1 290.1]  Denominator=[1 298.8]
  Trigonometric Function1 : Trigonometry
  V> pu : Gain  Gain=1/Vbase/sqrt(3)  SaturateOnIntegerOverflow=on  OutDataTypeStr=Inherit: Same as input  ParamDataTypeStr=Inherit: Same as input
  V> pu1 : Gain  Gain=sqrt(2)  SaturateOnIntegerOverflow=on  OutDataTypeStr=Inherit: Same as input  ParamDataTypeStr=Inherit: Same as input
  i : Outport
  wires:
  V> pu/1 -> PLL/1(v (pu)), V> pu1/1
  Real-Imag to Complex/1 -> Positive Sequence  current/1(V1(pu))
  PQ/1 -> Demux/1
  Demux/1 -> Real-Imag to Complex1/1
  Demux/2 -> -Q/1
  Real-Imag to Complex1/1 -> Positive Sequence  current/2(S_ext)
  Complex to Real-Imag1/1 -> Real-Imag to Complex/1
  Complex to Real-Imag1/2 -> Real-Imag to Complex/2
  Magnitude-Angle to Complex/1 -> Complex to Real-Imag1/1
  Constant/1 -> PLL/2(freq (pu))
  PLL/1(alpha (rad)) -> Magnitude-Angle to Complex/2
  Complex to Magnitude-Angle/2 -> Sum/2
  PLL/2(wt) -> Sum/1
  Sum/1 -> Trigonometric Function1/1
  Trigonometric Function1/1 -> Divide/2
  Complex to Magnitude-Angle/1 -> Divide/1
  RMS1/1 -> IC1/1
  V> pu1/1 -> RMS1/1
  v/1 -> IC2/1
  Positive Sequence  current/1(I1(A)) -> Break  Alg. Loop1/1(In)
  Break  Alg. Loop1/1(Out) -> Complex to Magnitude-Angle/1
  IC1/1 -> Magnitude-Angle to Complex/1
  IC2/1 -> V> pu/1
  Transfer Fcn1/1 -> Gain/1
  Gain/1 -> i/1
  Divide/1 -> Transfer Fcn1/1
  -Q/1 -> Real-Imag to Complex1/2

== system Feeder_1/SM_NG/Single-Phase Dynamic Load58/model ==
  v : Inport
  PQ : Inport  Port=2
  -Q : Gain  SaturateOnIntegerOverflow=on  OutDataTypeStr=Inherit: Same as input  ParamDataTypeStr=Inherit: Same as input
  Break  Alg. Loop1 : Subsystem
  Complex to Magnitude-Angle : ComplexToMagnitudeAngle
  Complex to Real-Imag1 : ComplexToRealImag
  Constant : Constant
  Demux : Demux  Outputs=2
  Divide : Product  Inputs=**
  Gain : Gain  Gain=1.0114
  IC1 : InitialCondition
  IC2 : InitialCondition
  Magnitude-Angle to Complex : MagnitudeAngleToComplex
  PLL : Subsystem  mask{freq=fnom}
      mask prompts: freq "Initial frequency (Hz)"
  Positive Sequence  current : Subsystem
  RMS1 : powerlib_meascontrol/Measurements/RMS  TrueRMS=on  Freq=fnom  RMSInit=1  Ts=0
  Real-Imag to Complex : RealImagToComplex
  Real-Imag to Complex1 : RealImagToComplex
  Sum : Sum
  Transfer Fcn1 : TransferFcn  Numerator=[1 290.1]  Denominator=[1 298.8]
  Trigonometric Function1 : Trigonometry
  V> pu : Gain  Gain=1/Vbase/sqrt(3)  SaturateOnIntegerOverflow=on  OutDataTypeStr=Inherit: Same as input  ParamDataTypeStr=Inherit: Same as input
  V> pu1 : Gain  Gain=sqrt(2)  SaturateOnIntegerOverflow=on  OutDataTypeStr=Inherit: Same as input  ParamDataTypeStr=Inherit: Same as input
  i : Outport
  wires:
  V> pu/1 -> PLL/1(v (pu)), V> pu1/1
  Real-Imag to Complex/1 -> Positive Sequence  current/1(V1(pu))
  PQ/1 -> Demux/1
  Demux/1 -> Real-Imag to Complex1/1
  Demux/2 -> -Q/1
  Real-Imag to Complex1/1 -> Positive Sequence  current/2(S_ext)
  Complex to Real-Imag1/1 -> Real-Imag to Complex/1
  Complex to Real-Imag1/2 -> Real-Imag to Complex/2
  Magnitude-Angle to Complex/1 -> Complex to Real-Imag1/1
  Constant/1 -> PLL/2(freq (pu))
  PLL/1(alpha (rad)) -> Magnitude-Angle to Complex/2
  Complex to Magnitude-Angle/2 -> Sum/2
  PLL/2(wt) -> Sum/1
  Sum/1 -> Trigonometric Function1/1
  Trigonometric Function1/1 -> Divide/2
  Complex to Magnitude-Angle/1 -> Divide/1
  RMS1/1 -> IC1/1
  V> pu1/1 -> RMS1/1
  v/1 -> IC2/1
  Positive Sequence  current/1(I1(A)) -> Break  Alg. Loop1/1(In)
  Break  Alg. Loop1/1(Out) -> Complex to Magnitude-Angle/1
  IC1/1 -> Magnitude-Angle to Complex/1
  IC2/1 -> V> pu/1
  Transfer Fcn1/1 -> Gain/1
  Gain/1 -> i/1
  Divide/1 -> Transfer Fcn1/1
  -Q/1 -> Real-Imag to Complex1/2

== system Feeder_1/SM_NG/Single-Phase Dynamic Load59/model ==
  v : Inport
  PQ : Inport  Port=2
  -Q : Gain  SaturateOnIntegerOverflow=on  OutDataTypeStr=Inherit: Same as input  ParamDataTypeStr=Inherit: Same as input
  Break  Alg. Loop1 : Subsystem
  Complex to Magnitude-Angle : ComplexToMagnitudeAngle
  Complex to Real-Imag1 : ComplexToRealImag
  Constant : Constant
  Demux : Demux  Outputs=2
  Divide : Product  Inputs=**
  Gain : Gain  Gain=1.0114
  IC1 : InitialCondition
  IC2 : InitialCondition
  Magnitude-Angle to Complex : MagnitudeAngleToComplex
  PLL : Subsystem  mask{freq=fnom}
      mask prompts: freq "Initial frequency (Hz)"
  Positive Sequence  current : Subsystem
  RMS1 : powerlib_meascontrol/Measurements/RMS  TrueRMS=on  Freq=fnom  RMSInit=1  Ts=0
  Real-Imag to Complex : RealImagToComplex
  Real-Imag to Complex1 : RealImagToComplex
  Sum : Sum
  Transfer Fcn1 : TransferFcn  Numerator=[1 290.1]  Denominator=[1 298.8]
  Trigonometric Function1 : Trigonometry
  V> pu : Gain  Gain=1/Vbase/sqrt(3)  SaturateOnIntegerOverflow=on  OutDataTypeStr=Inherit: Same as input  ParamDataTypeStr=Inherit: Same as input
  V> pu1 : Gain  Gain=sqrt(2)  SaturateOnIntegerOverflow=on  OutDataTypeStr=Inherit: Same as input  ParamDataTypeStr=Inherit: Same as input
  i : Outport
  wires:
  V> pu/1 -> PLL/1(v (pu)), V> pu1/1
  Real-Imag to Complex/1 -> Positive Sequence  current/1(V1(pu))
  PQ/1 -> Demux/1
  Demux/1 -> Real-Imag to Complex1/1
  Demux/2 -> -Q/1
  Real-Imag to Complex1/1 -> Positive Sequence  current/2(S_ext)
  Complex to Real-Imag1/1 -> Real-Imag to Complex/1
  Complex to Real-Imag1/2 -> Real-Imag to Complex/2
  Magnitude-Angle to Complex/1 -> Complex to Real-Imag1/1
  Constant/1 -> PLL/2(freq (pu))
  PLL/1(alpha (rad)) -> Magnitude-Angle to Complex/2
  Complex to Magnitude-Angle/2 -> Sum/2
  PLL/2(wt) -> Sum/1
  Sum/1 -> Trigonometric Function1/1
  Trigonometric Function1/1 -> Divide/2
  Complex to Magnitude-Angle/1 -> Divide/1
  RMS1/1 -> IC1/1
  V> pu1/1 -> RMS1/1
  v/1 -> IC2/1
  Positive Sequence  current/1(I1(A)) -> Break  Alg. Loop1/1(In)
  Break  Alg. Loop1/1(Out) -> Complex to Magnitude-Angle/1
  IC1/1 -> Magnitude-Angle to Complex/1
  IC2/1 -> V> pu/1
  Transfer Fcn1/1 -> Gain/1
  Gain/1 -> i/1
  Divide/1 -> Transfer Fcn1/1
  -Q/1 -> Real-Imag to Complex1/2

== system Feeder_1/SM_NG/Single-Phase Dynamic Load60/model ==
  v : Inport
  PQ : Inport  Port=2
  -Q : Gain  SaturateOnIntegerOverflow=on  OutDataTypeStr=Inherit: Same as input  ParamDataTypeStr=Inherit: Same as input
  Break  Alg. Loop1 : Subsystem
  Complex to Magnitude-Angle : ComplexToMagnitudeAngle
  Complex to Real-Imag1 : ComplexToRealImag
  Constant : Constant
  Demux : Demux  Outputs=2
  Divide : Product  Inputs=**
  Gain : Gain  Gain=1.0114
  IC1 : InitialCondition
  IC2 : InitialCondition
  Magnitude-Angle to Complex : MagnitudeAngleToComplex
  PLL : Subsystem  mask{freq=fnom}
      mask prompts: freq "Initial frequency (Hz)"
  Positive Sequence  current : Subsystem
  RMS1 : powerlib_meascontrol/Measurements/RMS  TrueRMS=on  Freq=fnom  RMSInit=1  Ts=0
  Real-Imag to Complex : RealImagToComplex
  Real-Imag to Complex1 : RealImagToComplex
  Sum : Sum
  Transfer Fcn1 : TransferFcn  Numerator=[1 290.1]  Denominator=[1 298.8]
  Trigonometric Function1 : Trigonometry
  V> pu : Gain  Gain=1/Vbase/sqrt(3)  SaturateOnIntegerOverflow=on  OutDataTypeStr=Inherit: Same as input  ParamDataTypeStr=Inherit: Same as input
  V> pu1 : Gain  Gain=sqrt(2)  SaturateOnIntegerOverflow=on  OutDataTypeStr=Inherit: Same as input  ParamDataTypeStr=Inherit: Same as input
  i : Outport
  wires:
  V> pu/1 -> PLL/1(v (pu)), V> pu1/1
  Real-Imag to Complex/1 -> Positive Sequence  current/1(V1(pu))
  PQ/1 -> Demux/1
  Demux/1 -> Real-Imag to Complex1/1
  Demux/2 -> -Q/1
  Real-Imag to Complex1/1 -> Positive Sequence  current/2(S_ext)
  Complex to Real-Imag1/1 -> Real-Imag to Complex/1
  Complex to Real-Imag1/2 -> Real-Imag to Complex/2
  Magnitude-Angle to Complex/1 -> Complex to Real-Imag1/1
  Constant/1 -> PLL/2(freq (pu))
  PLL/1(alpha (rad)) -> Magnitude-Angle to Complex/2
  Complex to Magnitude-Angle/2 -> Sum/2
  PLL/2(wt) -> Sum/1
  Sum/1 -> Trigonometric Function1/1
  Trigonometric Function1/1 -> Divide/2
  Complex to Magnitude-Angle/1 -> Divide/1
  RMS1/1 -> IC1/1
  V> pu1/1 -> RMS1/1
  v/1 -> IC2/1
  Positive Sequence  current/1(I1(A)) -> Break  Alg. Loop1/1(In)
  Break  Alg. Loop1/1(Out) -> Complex to Magnitude-Angle/1
  IC1/1 -> Magnitude-Angle to Complex/1
  IC2/1 -> V> pu/1
  Transfer Fcn1/1 -> Gain/1
  Gain/1 -> i/1
  Divide/1 -> Transfer Fcn1/1
  -Q/1 -> Real-Imag to Complex1/2
